simulink model "EE498_rafetkavak_termproject_part1_platooning_controlsystemdesign_simulinkmodel"  (R2019b)
settings: Solver=VariableStepAuto  StartTime=0.0  StopTime=10.0  RelTol=1e-3
libraries: cstblocks x3
settings Model: Creator=rafet  LastModifiedBy=rafet

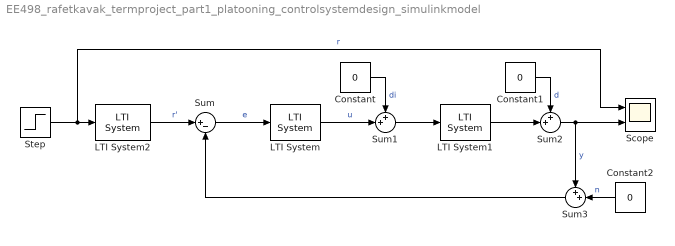
== system EE498_rafetkavak_termproject_part1_platooning_controlsystemdesign_simulinkmodel ==
  Constant : Constant  Value=0
  Constant1 : Constant  Value=0
  Constant2 : Constant  Value=0
  LTI System : cstblocks/LTI System  sys=C5  IC=[]
  LTI System1 : cstblocks/LTI System  sys=G  IC=[]
  LTI System2 : cstblocks/LTI System  sys=F  IC=[]
  Scope : Scope  NumInputPorts=2
  Step : Step  SampleTime=0
  Sum : Sum  Inputs=|+-
  Sum1 : Sum  Inputs=++|
  Sum2 : Sum  Inputs=++|
  Sum3 : Sum  Inputs=++|
  wires:
  LTI System1/1 -> Sum2/2
  Sum1/1 -> LTI System1/1
  LTI System/1 -> Sum1/2  "u"
  Sum/1 -> LTI System/1  "e"
  LTI System2/1 -> Sum/1  "r'"
  Sum2/1 -> Scope/2, Sum3/1  "y"
  Sum3/1 -> Sum/2
  Step/1 -> Scope/1, LTI System2/1  "r"
  Constant/1 -> Sum1/1  "di"
  Constant1/1 -> Sum2/1  "d"
  Constant2/1 -> Sum3/2  "n"
